simulink model "A2_2_P_angle"  (Simulink 7.4)
settings: Solver=FixedStepDiscrete  StartTime=0.0  StopTime=10  RelTol=1e-3
undefined symbols (not defined in the file): Kp
libraries: DCmotor_library x1
settings Model: Creator=Natalia  LastModifiedBy=ma
settings DebuggingCC: StrictBusMsg=ErrorLevel1
settings HardwareCC: ProdIntDivRoundTo=Zero  ProdEndianess=LittleEndian  ProdHWDeviceType=Generic->32-bit x86 compatible
settings RTWCC: SystemTargetFile=rtwin.tlc  TemplateMakefile=rtwin.tmf  Description=Real-Time Windows Target  ProcessScript=rtwin_make_rtw_hook  RTWCompilerOptimization=On
settings CodeAppCC: MaxIdLength=95  CustomSymbolStrType=$N$R$M_T
settings TargetCC: TargetLibSuffix=_rtwin.lib  TargetPreCompLibLocation=C:\Program Files\MATLAB\R2012b\toolbox\rtw\targets\rtwin\lib\win64  TargetFunctionLibrary=ANSI_C  IsPILTarget=off  MatFileLogging=on  EnableShiftOperators=on
settings CustomProperty: DataType=string  Value=C:/PROGRA~1/MATLAB/R2012b/toolbox/rtw/targets/rtwin

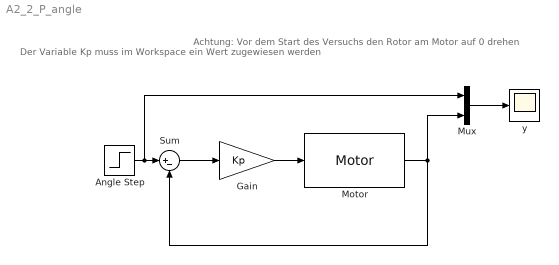
== system A2_2_P_angle ==
  note: Der Variable Kp
      | muss im Workspace ein
      | Wert zugewiesen werden
  note: Achtung:
      | Vor dem Start des Versuchs
      | den Rotor am Motor auf 0 drehen
  Angle Step : Step  After=2*pi  SampleTime=0.01
  Gain : Gain  Gain=Kp
  Motor : DCmotor_library/Motor  motoridinput=8  name_signal=Angle  ts=10
  Mux : Mux  Inputs=2
  Sum : Sum  Inputs=|+-
  y : Scope
      settings: YMin=-4  YMax=20
  wires:
  Angle Step/1 -> Mux/1, Sum/1
  Sum/1 -> Gain/1
  Motor/1 -> Mux/2, Sum/2
  Gain/1 -> Motor/1
  Mux/1 -> y/1
